simulink model "eg2_5"  (R2014a)
settings: Solver=ode45  StartTime=0.0  StopTime=10.0  RelTol=1e-3
settings Model: Creator=tzb  LastModifiedBy=tzb

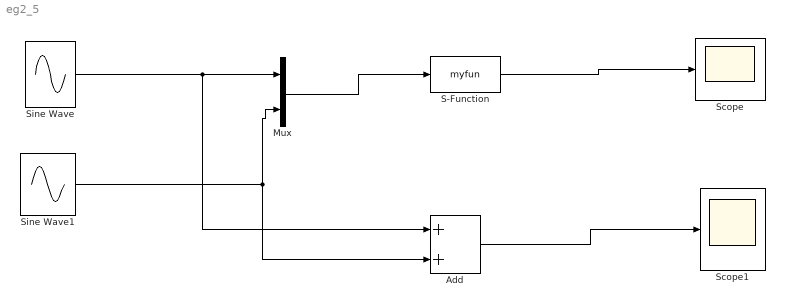
== system eg2_5 ==
  Add : Sum
  Mux : Mux  Inputs=2
  S-Function : S-Function  FunctionName=myfun  EnableBusSupport=off
  Scope : Scope
  Scope1 : Scope
  Sine Wave : Sin  SampleTime=0
  Sine Wave1 : Sin  Frequency=2  Phase=pi/2  SampleTime=0
  wires:
  Sine Wave/1 -> Add/1, Mux/1
  Mux/1 -> S-Function/1
  Sine Wave1/1 -> Add/2, Mux/2
  S-Function/1 -> Scope/1
  Add/1 -> Scope1/1
